simulink model "Long_Accel_Track"  (R2020b)
settings: Solver=VariableStepAuto  StartTime=0.0  StopTime=60  RelTol=1e-3
values from neighbouring files (symbols this model uses):
  Accreq_valueY = [-6 -5.8 -5.6 -5.4 -5.2 -5 -4.8 -4.6 -4.4 -4.2 -4 -3.8 ... (53 elements, 1x53)]    [Accreq_valueY.mat]    (also in make_calibrate_table.m = [-6:0.2:-0.1,0.1:0.2:4.5])
  Openness_valueZ = [-100 -100 -100 -100 -96.0255330412 -92.5475086479 -89.5294536846 -86.0415379146 -82.7286102821 -79.845577645 -76.1908087806 -72.5393369095 ... (1643 elements, 53x31)]    [Openness_valueZ.mat]    (also in make_calibrate_table.m = zeros(length(Accreq_valueY), length(Vehspd_valueX)))
  Vehspd_valueX = [0 4 8 12 16 20 24 28 32 36 40 44 ... (31 elements, 1x31)]    [Vehspd_valueX.mat]    (also in make_calibrate_table.m = 0:4:120)
libraries: Solver_SF x1, pid_lib x1
settings Model: Creator=cv  LastModifiedBy=cv

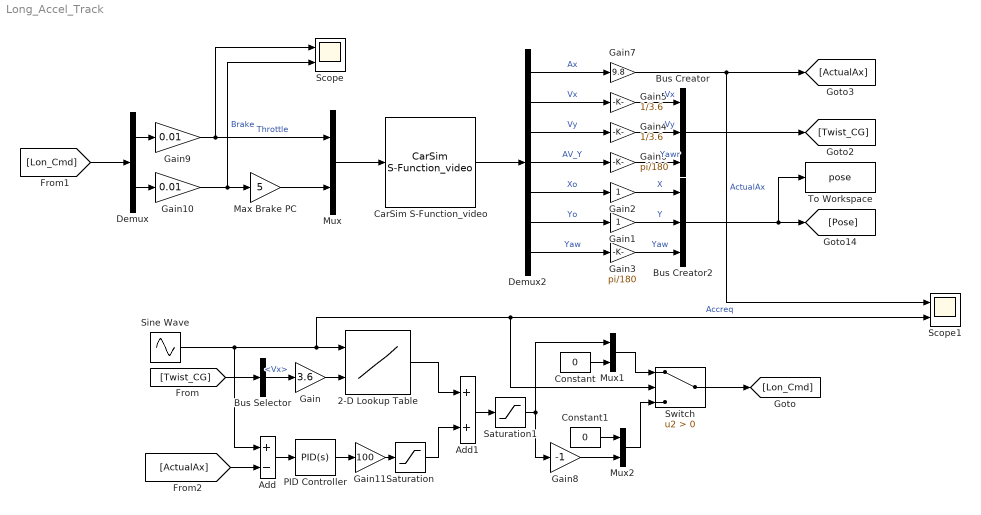
== system Long_Accel_Track ==
  2-D Lookup Table : Lookup_n-D  BreakpointsForDimension1=Accreq_valueY  BreakpointsForDimension2=Vehspd_valueX  Table=Openness_valueZ  InternalRulePriority=Speed  RndMeth=Simplest  InputSameDT=on
      settings: InputPortMap=u0,u1
  Add : Sum  Inputs=+-
  Add1 : Sum
  Bus Creator : BusCreator  Inputs=3
  Bus Creator2 : BusCreator  Inputs=3
  Bus Selector : BusSelector  OutputSignals=Vx
  CarSim S-Function_video : Solver_SF/CarSim S-Function_video  Priority=1  SIMFILE=accel_track.sim
      settings: SourceProductName=CarSim S-Function
  Constant : Constant  Value=0
  Constant1 : Constant  Value=0
  Demux : Demux  Outputs=2
  Demux2 : Demux  Outputs=7
  Gain : Gain  Gain=3.6
  Gain1 : Gain
  Gain10 : Gain  Gain=0.01
  Gain11 : Gain  Gain=100
  Gain2 : Gain
  Gain3 : Gain  Gain=pi/180
  Gain4 : Gain  Gain=1/3.6
  Gain5 : Gain  Gain=1/3.6
  Gain6 : Gain  Gain=pi/180
  Gain7 : Gain  Gain=9.8
  Gain8 : Gain  Gain=-1
  Gain9 : Gain  Gain=0.01
  Max Brake PC : Gain  Gain=5
  Mux : Mux  Inputs=2
  Mux1 : Mux  Inputs=2
  Mux2 : Mux  Inputs=2
  PID Controller : pid_lib/PID Controller  Controller=PID  Form=Parallel  TimeDomain=Continuous-time  UseExternalTs=off  SampleTime=-1  IntegratorMethod=Forward Euler  FilterMethod=Forward Euler  ControllerParametersSource=internal  P=0.55  I=0.015  D=0  UseFilter=on  N=100  TunerSelectOption=Transfer Function Based (PID Tuner App)  InitialConditionSource=internal  InitialConditionForIntegrator=0  InitialConditionForFilter=0  DifferentiatorICPrevScaledInput=0  ExternalReset=none  TrackingMode=off  Kt=1  LimitOutput=off  SatLimitsSource=internal  UpperSaturationLimit=inf  LowerSaturationLimit=-inf  LinearizeAsGain=on  AntiWindupMode=none  Kb=1  POutMin=[]  POutMax=[]  IOutMin=[]  IOutMax=[]  DOutMin=[]  DOutMax=[]  NOutMin=[]  NOutMax=[]  SumOutMin=[]  SumOutMax=[]  SaturationOutMin=[]  SaturationOutMax=[]  PParamMin=[]  PParamMax=[]  IParamMin=[]  IParamMax=[]  DParamMin=[]  DParamMax=[]  NParamMin=[]  NParamMax=[]  KbParamMin=[]  KbParamMax=[]  KtParamMin=[]  KtParamMax=[]  KbOutMin=[]  KbOutMax=[]  KtOutMin=[]  KtOutMax=[]  IntegratorOutMin=[]  IntegratorOutMax=[]  FilterOutMin=[]  FilterOutMax=[]  SumI1OutMin=[]  SumI1OutMax=[]  SumI2OutMin=[]  SumI2OutMax=[]  SumI3OutMin=[]  SumI3OutMax=[]  SumI4OutMin=[]  SumI4OutMax=[]  SumDOutMin=[]  SumDOutMax=[]  DifferentiatorOutMin=[]  DifferentiatorOutMax=[]  FilterDiffOutCoefMin=[]  FilterDiffOutCoefMax=[]  ReciprocalOutMin=[]  ReciprocalOutMax=[]  SumDenOutMin=[]  SumDenOutMax=[]  SumNumOutMin=[]  SumNumOutMax=[]  DivideOutMin=[]  DivideOutMax=[]  UdiffTsProdOutMin=[]  UdiffTsProdOutMax=[]  NTsProdOutMin=[]  NTsProdOutMax=[]  UintegralTsProdOutMin=[]  UintegralTsProdOutMax=[]  UngainTsProdOutMin=[]  UngainTsProdOutMax=[]  IntegratorContinuousStateAttributes=''  IntegratorStateMustResolveToSignalObject=off  IntegratorRTWStateStorageClass=Auto  FilterContinuousStateAttributes=''  FilterStateMustResolveToSignalObject=off  FilterRTWStateStorageClass=Auto  ParallelPVariant=InternalParameters  IdealPVariant=Disabled  IVariant=InternalParameters  DVariant=InternalParameters  IntegratorVariant=Continuous  SatVariant=Disabled  AWVariant=Passthrough  PCopyVariant=Disabled  TRVariant=Disabled  FdbkBlocksVariant=Forward  IdealPFdbkVariant=Disabled  SatFdbkVariant=Disabled  DerivativeFilterVariant=ContFilter  NVariant=InternalParameters  NCopyVariant=Disabled  FilterICVariant=InternalICsFilter  IntegratorICVariant=InternalICs  ExternalResetVariant=Disabled  TRSumVariant=Passthrough  SumFdbkVariant=Disabled  SumVariant=Sum_PID  TsampFilterVariant=InternalTs  TsampNgainVariant=Passthrough  TsampIntegralVariant=Passthrough  ExternalSaturationOutDataTypeStr=Inherit: Same as second input
  Saturation : Saturate  UpperLimit=50  LowerLimit=-50
  Saturation1 : Saturate  UpperLimit=100  LowerLimit=-100
  Scope : Scope  NumInputPorts=2
  Scope1 : Scope  NumInputPorts=2
  Sine Wave : Sin  Amplitude=4.0  Frequency=2*pi/15  SampleTime=0
  Switch : Switch  Criteria=u2 > Threshold
  To Workspace : ToWorkspace  VariableName=pose  SaveFormat=Timeseries  SampleTime=-1
  wires:
  Mux/1 -> CarSim S-Function_video/1
  CarSim S-Function_video/1 -> Demux2/1
  Gain9/1 -> Mux/1, Scope/1  "Throttle"
  Gain10/1 -> Scope/2, Max Brake PC/1  "Brake"
  Max Brake PC/1 -> Mux/2
  Gain6/1 -> Bus Creator/3  "Yawr"
  Demux2/6 -> Gain1/1  "Yo"
  Gain2/1 -> Bus Creator2/1  "X"
  Demux2/1 -> Gain7/1  "Ax"
  Bus Creator2/1 -> To Workspace/1, [Pose]
  Gain3/1 -> Bus Creator2/3  "Yaw"
  Gain7/1 -> Scope1/1, [ActualAx]  "ActualAx"
  Demux2/4 -> Gain6/1  "AV_Y"
  Gain5/1 -> Bus Creator/1  "Vx"
  Demux2/2 -> Gain5/1  "Vx"
  Gain1/1 -> Bus Creator2/2  "Y"
  Demux2/3 -> Gain4/1  "Vy"
  Demux2/7 -> Gain3/1  "Yaw"
  Bus Creator/1 -> [Twist_CG]
  Gain4/1 -> Bus Creator/2  "Vy"
  Demux2/5 -> Gain2/1  "Xo"
  Sine Wave/1 -> Add/1, Switch/2, Scope1/2, 2-D Lookup Table/1  "Accreq"
  [Twist_CG] -> Bus Selector/1
  Bus Selector/1 -> Gain/1  "<Vx>"
  Gain/1 -> 2-D Lookup Table/2
  Constant/1 -> Mux1/2
  Mux1/1 -> Switch/1
  Mux2/1 -> Switch/3
  Constant1/1 -> Mux2/1
  Gain8/1 -> Mux2/2
  Switch/1 -> [Lon_Cmd]
  [Lon_Cmd] -> Demux/1
  Demux/1 -> Gain9/1
  Demux/2 -> Gain10/1
  Add/1 -> PID Controller/1
  [ActualAx] -> Add/2
  2-D Lookup Table/1 -> Add1/1
  Saturation/1 -> Add1/2
  PID Controller/1 -> Gain11/1
  Gain11/1 -> Saturation/1
  Add1/1 -> Saturation1/1
  Saturation1/1 -> Gain8/1, Mux1/1
